simulink model "dp_mod_model_Matlab2022b"  (R2022b)
settings: Solver=ode45  StartTime=0.0  StopTime=sim_time  RelTol=1e-3  EnableMultiTasking=on
values from neighbouring files (symbols this model uses):
  fc = 40    [sim_dp_mod_model.m]
  fmod = 20    [sim_dp_mod_model.m]
  fsc = 96    [sim_dp_mod_model.m]
  im_am = 0    [sim_dp_mod_model.m]
  im_fm = 500    [sim_dp_mod_model.m]
libraries: dspsrcs4 x1
settings Model: Creator=jvalls  LastModifiedBy=jvc
settings SolverCC: AlgebraicLoopSolver=TrustRegion
settings DataIOCC: LimitDataPoints=on  SaveFormat=Array  ReturnWorkspaceOutputs=off
settings OptimizationCC: ReuseModelBlockBuffer=on  LifeSpan=inf
settings DebuggingCC: SolverPrmCheckMsg=warning  UnconnectedInputMsg=warning  UnconnectedOutputMsg=warning  UnconnectedLineMsg=warning  SFUnexpectedBacktrackingDiag=warning  SFNoUnconditionalDefaultTransitionDiag=warning  SFExecutionAtInitializationDiag=none  ArithmeticOperatorsInVariantConditions=warning
settings HardwareCC: ProdBitPerPointer=32  ProdBitPerSizeT=32  ProdBitPerPtrDiffT=32  ProdLargestAtomicFloat=None  ProdIntDivRoundTo=Undefined  ProdEndianess=Unspecified  ProdWordSize=32  ProdHWDeviceType=32-bit Generic
settings ModelReferenceCC: EnableRefExpFcnMdlSchedulingChecks=on  PropagateSignalLabelsOutOfModel=off
settings SFSimCC: SimUseLocalCustomCode=off  CustomCodeUndefinedFunction=UseInterfaceOnly
settings RTWCC: RTWUseLocalCustomCode=off
settings CodeAppCC: StateflowObjectComments=on
settings GRTTargetCC: TargetLangStandard=C89/C90 (ANSI)
settings ConfigComp: CovMetricSettings=dw  CovSaveCumulativeToWorkspaceVar=on  CovSaveSingleToWorkspaceVar=on  CovExternalEMLEnable=off  CovSFcnEnable=off

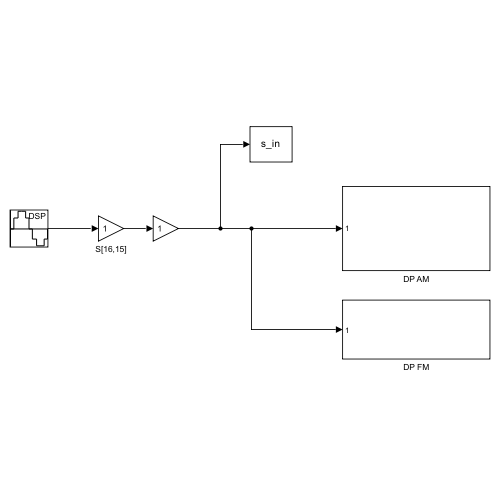
[thumbnail: Simulink's stored preview of the top-level diagram]
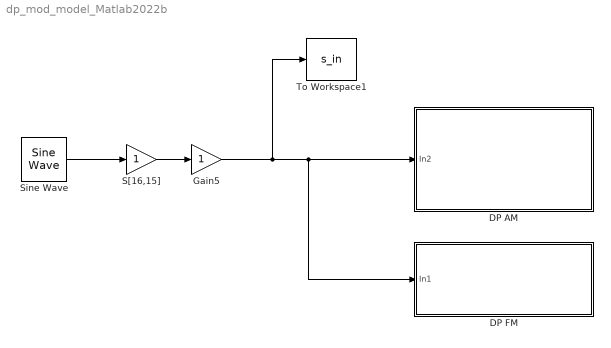
== system dp_mod_model_Matlab2022b ==
  DP AM : Subsystem
  DP FM : Subsystem
  Gain5 : Gain  OutDataTypeStr=double
  S[16,15] : Gain  OutDataTypeStr=fixdt(1,16,15)  RndMeth=Nearest
  Sine Wave : dspsrcs4/Sine Wave  Amplitude=1-2^-15  Frequency=fmod/1000  Phase=-pi/40  SampleMode=Discrete  OutComplex=Real  CompMethod=Trigonometric fcn  TableSize=Speed  SampleTime=1/fsc  SamplesPerFrame=1  ResetState=Restart at time zero  OutputFrames=on  dataType=double  wordLen=16  udDataType=sfix(16)  fracBitsMode=Best precision  numFracBits=15  OutDataTypeStr=double  LastOutDataTypeStr=double
  To Workspace1 : ToWorkspace  VariableName=s_in  SampleTime=-1
      settings: Save2DSignal=2-D array (concatenate along first dimension)
  wires:
  Sine Wave/1 -> S[16,15]/1
  S[16,15]/1 -> Gain5/1
  Gain5/1 -> To Workspace1/1, DP FM/1(In1), DP AM/1(In2)

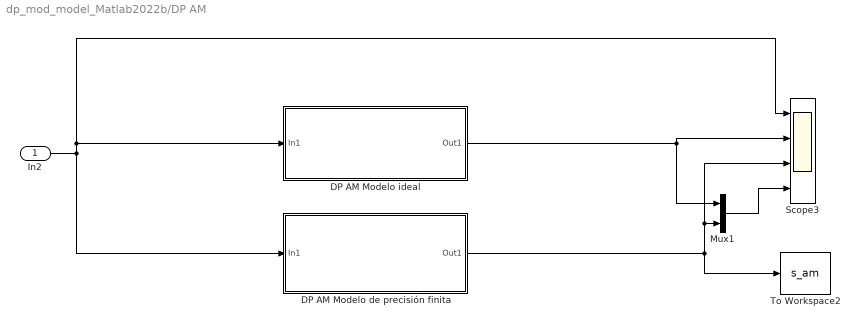
== system dp_mod_model_Matlab2022b/DP AM ==
  In2 : Inport
  DP AM Modelo de precisión finita : Subsystem
  DP AM Modelo ideal : Subsystem
  Mux1 : Mux  Inputs=2
  Scope3 : Scope  NumInputPorts=4
  To Workspace2 : ToWorkspace  VariableName=s_am  SampleTime=-1
      settings: Save2DSignal=2-D array (concatenate along first dimension)
  wires:
  Mux1/1 -> Scope3/4
  DP AM Modelo de precisión finita/1(Out1) -> Scope3/3, Mux1/2, To Workspace2/1
  DP AM Modelo ideal/1(Out1) -> Scope3/2, Mux1/1
  In2/1 -> Scope3/1, DP AM Modelo ideal/1(In1), DP AM Modelo de precisión finita/1(In1)

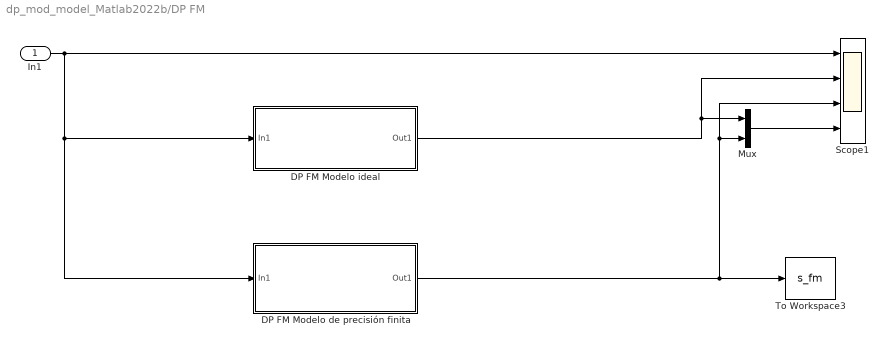
== system dp_mod_model_Matlab2022b/DP FM ==
  In1 : Inport
  DP FM Modelo de precisión finita : Subsystem
  DP FM Modelo ideal : Subsystem
  Mux : Mux  Inputs=2
  Scope1 : Scope  NumInputPorts=4
  To Workspace3 : ToWorkspace  VariableName=s_fm  SampleTime=-1
      settings: Save2DSignal=2-D array (concatenate along first dimension)
  wires:
  In1/1 -> Scope1/1, DP FM Modelo de precisión finita/1(In1), DP FM Modelo ideal/1(In1)
  Mux/1 -> Scope1/4
  DP FM Modelo ideal/1(Out1) -> Scope1/2, Mux/1
  DP FM Modelo de precisión finita/1(Out1) -> Scope1/3, Mux/2, To Workspace3/1

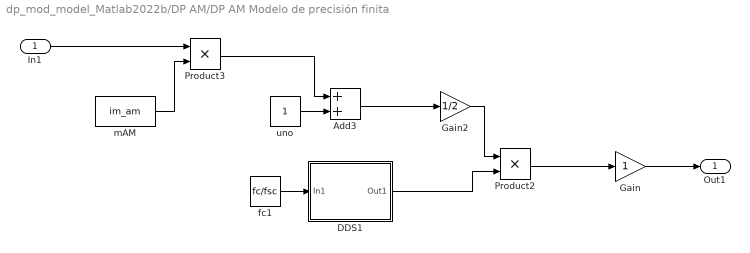
== system dp_mod_model_Matlab2022b/DP AM/DP AM Modelo de precisión finita ==
  In1 : Inport
  Add3 : Sum  AccumDataTypeStr=fixdt(1,17,15)  OutDataTypeStr=fixdt(1,17,15)
  DDS1 : Subsystem
  Gain : Gain  OutDataTypeStr=double
  Gain2 : Gain  Gain=1/2  OutDataTypeStr=fixdt(1,17,15)
  Product2 : Product  OutDataTypeStr=fixdt(1,16,15)
  Product3 : Product  OutDataTypeStr=fixdt(1,16,15)
  fc1 : Constant  Value=fc/fsc  OutDataTypeStr=fixdt(0,24,24)
  mAM : Constant  Value=im_am  OutDataTypeStr=fixdt(0,16,15)
  uno : Constant  OutDataTypeStr=fixdt(0,16,15)
  Out1 : Outport  VectorParamsAs1DForOutWhenUnconnected=off
  wires:
  uno/1 -> Add3/2
  Gain/1 -> Out1/1
  Product2/1 -> Gain/1
  Add3/1 -> Gain2/1
  Product3/1 -> Add3/1
  DDS1/1(Out1) -> Product2/2
  mAM/1 -> Product3/2
  In1/1 -> Product3/1
  fc1/1 -> DDS1/1(In1)
  Gain2/1 -> Product2/1

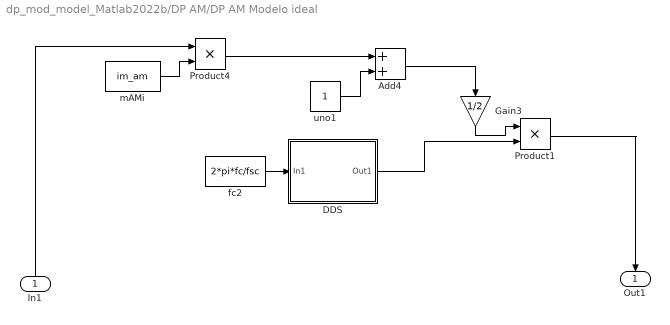
== system dp_mod_model_Matlab2022b/DP AM/DP AM Modelo ideal ==
  In1 : Inport
  Add4 : Sum
  DDS : Subsystem
  Gain3 : Gain  Gain=1/2  OutDataTypeStr=double
  Product1 : Product
  Product4 : Product
  fc2 : Constant  Value=2*pi*fc/fsc
  "mAMi " : Constant  Value=im_am
  uno1 : Constant
  Out1 : Outport  VectorParamsAs1DForOutWhenUnconnected=off
  wires:
  Product1/1 -> Out1/1
  Gain3/1 -> Product1/1
  In1/1 -> Product4/1
  Add4/1 -> Gain3/1
  uno1/1 -> Add4/2
  Product4/1 -> Add4/1
  "mAMi "/1 -> Product4/2
  DDS/1(Out1) -> Product1/2
  fc2/1 -> DDS/1(In1)

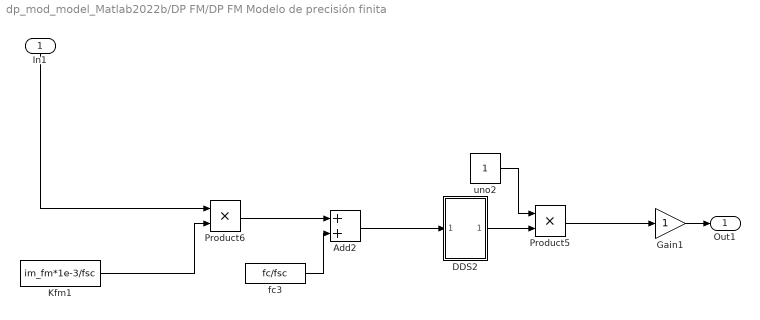
== system dp_mod_model_Matlab2022b/DP FM/DP FM Modelo de precisión finita ==
  In1 : Inport
  Add2 : Sum  AccumDataTypeStr=double  OutDataTypeStr=fixdt(1,24,24)
  DDS2 : Subsystem
  Gain1 : Gain  OutDataTypeStr=double
  Kfm1 : Constant  Value=im_fm*1e-3/fsc  OutDataTypeStr=fixdt(0,16,16)
  Product5 : Product  OutDataTypeStr=fixdt(1,16,15)
  Product6 : Product  OutDataTypeStr=fixdt(1,24,24)
  fc3 : Constant  Value=fc/fsc  OutDataTypeStr=fixdt(0,24,24)
  uno2 : Constant  OutDataTypeStr=fixdt(0,17,15)
  Out1 : Outport  VectorParamsAs1DForOutWhenUnconnected=off
  wires:
  Product6/1 -> Add2/1
  Add2/1 -> DDS2/1(In1)
  fc3/1 -> Add2/2
  In1/1 -> Product6/1
  uno2/1 -> Product5/1
  DDS2/1(Out1) -> Product5/2
  Kfm1/1 -> Product6/2
  Gain1/1 -> Out1/1
  Product5/1 -> Gain1/1

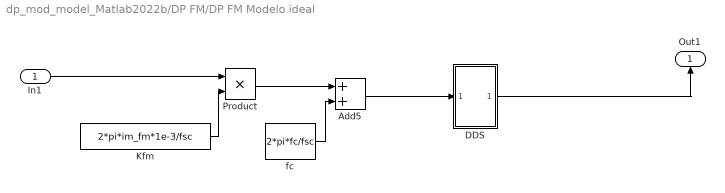
== system dp_mod_model_Matlab2022b/DP FM/DP FM Modelo ideal ==
  In1 : Inport
  Add5 : Sum
  DDS : Subsystem
  Kfm : Constant  Value=2*pi*im_fm*1e-3/fsc
  Product : Product
  fc : Constant  Value=2*pi*fc/fsc
  Out1 : Outport  VectorParamsAs1DForOutWhenUnconnected=off
  wires:
  DDS/1(Out1) -> Out1/1
  Add5/1 -> DDS/1(In1)
  Product/1 -> Add5/1
  In1/1 -> Product/1
  fc/1 -> Add5/2
  Kfm/1 -> Product/2

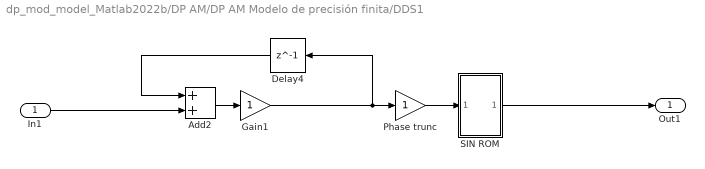
== system dp_mod_model_Matlab2022b/DP AM/DP AM Modelo de precisión finita/DDS1 ==
  In1 : Inport
  Add2 : Sum  AccumDataTypeStr=fixdt(0,24,24)  OutDataTypeStr=fixdt(0,24,24)  RndMeth=Convergent
  Delay4 : Delay  DelayLength=1
  Gain1 : Gain  OutDataTypeStr=double
  Phase trunc : Gain  OutDataTypeStr=fixdt(0,15,15)
  SIN ROM : Subsystem
  Out1 : Outport  VectorParamsAs1DForOutWhenUnconnected=off
  wires:
  Add2/1 -> Gain1/1
  Phase trunc/1 -> SIN ROM/1(In1)
  In1/1 -> Add2/2
  SIN ROM/1(Out1) -> Out1/1
  Gain1/1 -> Delay4/1, Phase trunc/1
  Delay4/1 -> Add2/1

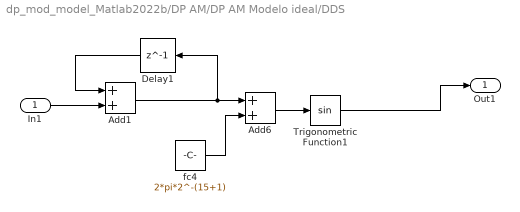
== system dp_mod_model_Matlab2022b/DP AM/DP AM Modelo ideal/DDS ==
  In1 : Inport
  Add1 : Sum
  Add6 : Sum
  Delay1 : Delay  DelayLength=1
  Trigonometric Function1 : Trigonometry
  fc4 : Constant  Value=2*pi*2^-(15+1)
  Out1 : Outport  VectorParamsAs1DForOutWhenUnconnected=off
  wires:
  Trigonometric Function1/1 -> Out1/1
  Add6/1 -> Trigonometric Function1/1
  Add1/1 -> Delay1/1, Add6/1
  In1/1 -> Add1/2
  fc4/1 -> Add6/2
  Delay1/1 -> Add1/1

== system dp_mod_model_Matlab2022b/DP FM/DP FM Modelo de precisión finita/DDS2 ==
  In1 : Inport
  Add8 : Sum  AccumDataTypeStr=fixdt(0,24,24)  OutDataTypeStr=fixdt(0,24,24)  RndMeth=Convergent
  Delay2 : Delay  DelayLength=1
  Phase trunc : Gain  OutDataTypeStr=fixdt(0,15,15)
  SIN ROM : Subsystem
  Out1 : Outport  VectorParamsAs1DForOutWhenUnconnected=off
  wires:
  Phase trunc/1 -> SIN ROM/1(In1)
  Add8/1 -> Phase trunc/1, Delay2/1
  SIN ROM/1(Out1) -> Out1/1
  In1/1 -> Add8/2
  Delay2/1 -> Add8/1

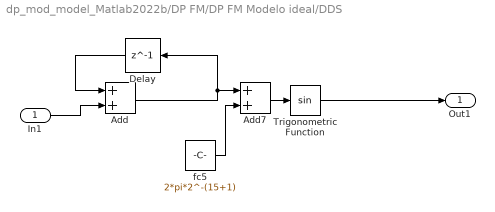
== system dp_mod_model_Matlab2022b/DP FM/DP FM Modelo ideal/DDS ==
  In1 : Inport
  Add : Sum
  Add7 : Sum
  Delay : Delay  DelayLength=1
  Trigonometric Function : Trigonometry
  fc5 : Constant  Value=2*pi*2^-(15+1)
  Out1 : Outport  VectorParamsAs1DForOutWhenUnconnected=off
  wires:
  Trigonometric Function/1 -> Out1/1
  fc5/1 -> Add7/2
  In1/1 -> Add/2
  Add/1 -> Add7/1, Delay/1
  Add7/1 -> Trigonometric Function/1
  Delay/1 -> Add/1

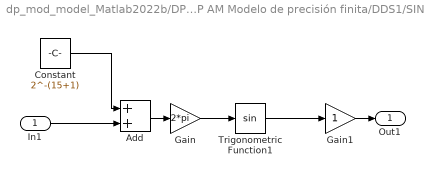
== system dp_mod_model_Matlab2022b/DP AM/DP AM Modelo de precisión finita/DDS1/SIN ROM ==
  In1 : Inport
  Add : Sum
  Constant : Constant  Value=2^-(15+1)
  Gain : Gain  Gain=2*pi
  Gain1 : Gain  OutDataTypeStr=fixdt(1,16,15)  RndMeth=Round  SaturateOnIntegerOverflow=on
  Trigonometric Function1 : Trigonometry
  Out1 : Outport  VectorParamsAs1DForOutWhenUnconnected=off
  wires:
  Add/1 -> Gain/1
  In1/1 -> Add/2
  Constant/1 -> Add/1
  Gain1/1 -> Out1/1
  Trigonometric Function1/1 -> Gain1/1
  Gain/1 -> Trigonometric Function1/1

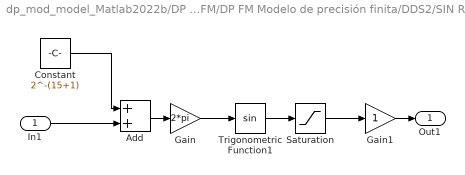
== system dp_mod_model_Matlab2022b/DP FM/DP FM Modelo de precisión finita/DDS2/SIN ROM ==
  In1 : Inport
  Add : Sum
  Constant : Constant  Value=2^-(15+1)
  Gain : Gain  Gain=2*pi
  Gain1 : Gain  OutDataTypeStr=fixdt(1,16,15)  RndMeth=Round  SaturateOnIntegerOverflow=on
  Saturation : Saturate  UpperLimit=1-2^-15  LowerLimit=-(1-2^-15)
  Trigonometric Function1 : Trigonometry
  Out1 : Outport  VectorParamsAs1DForOutWhenUnconnected=off
  wires:
  Add/1 -> Gain/1
  In1/1 -> Add/2
  Constant/1 -> Add/1
  Gain1/1 -> Out1/1
  Trigonometric Function1/1 -> Saturation/1
  Gain/1 -> Trigonometric Function1/1
  Saturation/1 -> Gain1/1
